simulink model "multi_model"  (R2017b)
settings: Solver=FixedStepAuto  StartTime=0.0  StopTime=10  RelTol=1e-3
undefined symbols (not defined in the file or in its folder): deg, motor_state, rad, s
libraries: simulink x7, aerolibconvert2 x4, aerolibobsolete x1, aerolibatmos2 x1, aerolibanimutils x1, aerolibnav x1
settings Model: SimulationMode=accelerator  Creator=ADAM  LastModifiedBy=moneu
settings DataIOCC: ExternalInput=initial_in  FinalStateName=final_state  InitialState=initial_state  LimitDataPoints=on  MaxDataPoints=1  LoadExternalInput=on  LoadInitialState=on  SaveFinalState=on  SaveFormat=Structure  SignalLoggingSaveFormat=ModelDataLogs  SignalLogging=off  DSMLogging=off  SaveTime=off  OutputSaveName=final_out  SignalLoggingName=model_out
settings OptimizationCC: ExpressionDepthLimit=2147483647  LifeSpan=inf
settings DebuggingCC: UnderspecifiedInitializationDetection=Classic  MergeDetectMultiDrivingBlocksExec=none  SolverPrmCheckMsg=warning  MultiTaskDSMMsg=warning  MultiTaskCondExecSysMsg=none  StateNameClashWarn=warning  StrictBusMsg=None  SFUnexpectedBacktrackingDiag=warning  SFNoUnconditionalDefaultTransitionDiag=warning  SFExecutionAtInitializationDiag=none
settings HardwareCC: ProdBitPerPointer=32  ProdBitPerSizeT=32  ProdBitPerPtrDiffT=32  ProdLargestAtomicFloat=None  ProdWordSize=32  ProdHWDeviceType=Generic->32-bit x86 compatible
settings ModelReferenceCC: UpdateModelReferenceTargets=AssumeUpToDate  CheckModelReferenceTargetMessage=none  PropagateSignalLabelsOutOfModel=off
settings RTWCC: SystemTargetFile=rtwin.tlc  TemplateMakefile=rtwin.tmf  Description=Real-Time Windows Target
settings CodeAppCC: MaxIdLength=95  StateflowObjectComments=on
settings TargetCC: TargetLibSuffix=_rtwin.lib  TargetPreCompLibLocation=C:\Program Files\MATLAB\R2013a\toolbox\rtw\targets\rtwin\lib\win64
settings ConfigComp: CovMetricSettings=dw  CovHtmlReporting=on  CovSaveCumulativeToWorkspaceVar=on  CovSaveSingleToWorkspaceVar=on  CovExternalEMLEnable=off

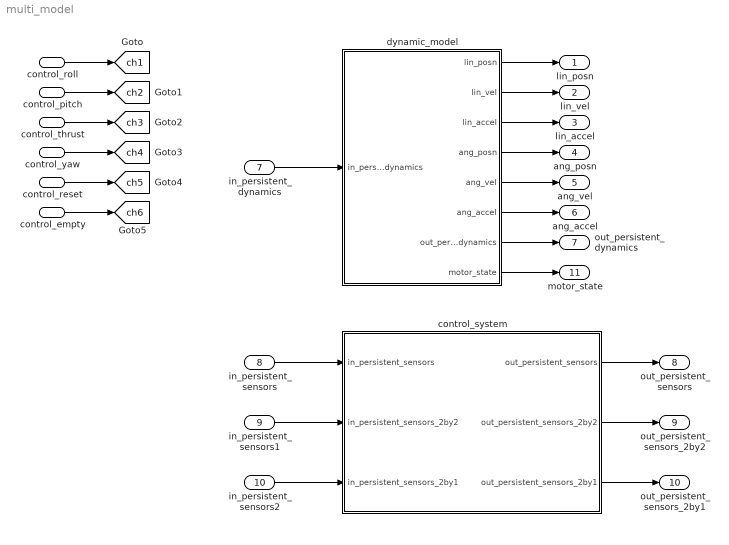
== system multi_model ==
  control_roll : Inport  PortDimensions=1
  control_pitch : Inport  Port=2  PortDimensions=1
  control_thrust : Inport  Port=3  PortDimensions=1
  control_yaw : Inport  Port=4  PortDimensions=1
  control_reset : Inport  Port=5  PortDimensions=1
  control_empty : Inport  Port=6  PortDimensions=1
  in_persistent_dynamics : Inport  Port=7  PortDimensions=1
  in_persistent_sensors : Inport  Port=8  PortDimensions=8
  in_persistent_sensors1 : Inport  Port=9  PortDimensions=[4 2]
  in_persistent_sensors2 : Inport  Port=10  PortDimensions=[2 2]
  control_system : Subsystem
  dynamic_model : Subsystem
  lin_posn : Outport
  lin_vel : Outport  Port=2
  lin_accel : Outport  Port=3
  ang_posn : Outport  Port=4
  ang_vel : Outport  Port=5
  ang_accel : Outport  Port=6
  out_persistent_dynamics : Outport  Port=7
  out_persistent_sensors : Outport  Port=8
  out_persistent_sensors_2by2 : Outport  Port=9
  out_persistent_sensors_2by1 : Outport  Port=10
  motor_state : Outport  Port=11
  tag scope: ch1=global, ch2=global, ch3=global, ch4=global, ch5=global, ch6=global
  wires:
  control_thrust/1 -> [ch3]
  control_pitch/1 -> [ch2]
  control_roll/1 -> [ch1]
  control_yaw/1 -> [ch4]
  control_reset/1 -> [ch5]
  control_empty/1 -> [ch6]
  dynamic_model/1(lin_posn) -> lin_posn/1
  dynamic_model/2(lin_vel) -> lin_vel/1
  dynamic_model/3(lin_accel) -> lin_accel/1
  dynamic_model/4(ang_posn) -> ang_posn/1
  dynamic_model/5(ang_vel) -> ang_vel/1
  dynamic_model/6(ang_accel) -> ang_accel/1
  dynamic_model/7(out_persistent_dynamics) -> out_persistent_dynamics/1
  control_system/1(out_persistent_sensors) -> out_persistent_sensors/1
  control_system/2(out_persistent_sensors_2by2) -> out_persistent_sensors_2by2/1
  control_system/3(out_persistent_sensors_2by1) -> out_persistent_sensors_2by1/1
  in_persistent_dynamics/1 -> dynamic_model/1(in_persistent_dynamics)
  in_persistent_sensors/1 -> control_system/1(in_persistent_sensors)
  in_persistent_sensors1/1 -> control_system/2(in_persistent_sensors_2by2)
  in_persistent_sensors2/1 -> control_system/3(in_persistent_sensors_2by1)
  dynamic_model/8(motor_state) -> motor_state/1

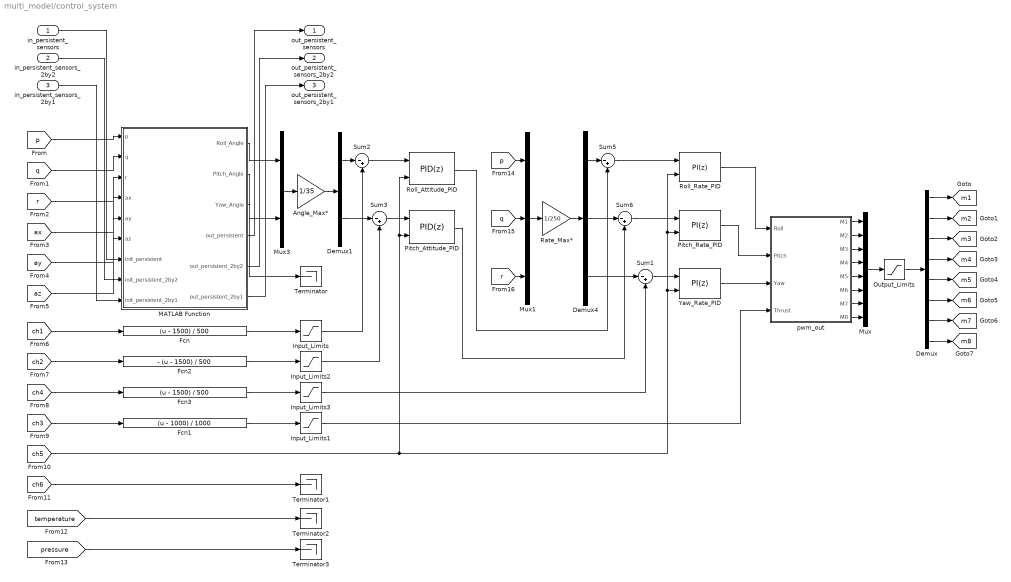
== system multi_model/control_system ==
  in_persistent_sensors : Inport
  in_persistent_sensors_2by2 : Inport  Port=2
  in_persistent_sensors_2by1 : Inport  Port=3
  Angle_Max* : Gain  Gain=1/35
  Demux : Demux  Outputs=8
  Demux1 : Demux  Outputs=2
  Demux4 : Demux  Outputs=3
  Fcn : Fcn  Expr=(u - 1500) / 500
  Fcn1 : Fcn  Expr=(u - 1000) / 1000
  Fcn2 : Fcn  Expr=- (u - 1500) / 500
  Fcn3 : Fcn  Expr=(u - 1500) / 500
  Input_Limits : Saturate  UpperLimit=1  LowerLimit=-1
  Input_Limits1 : Saturate  UpperLimit=1  LowerLimit=0
  Input_Limits2 : Saturate  UpperLimit=1  LowerLimit=-1
  Input_Limits3 : Saturate  UpperLimit=1  LowerLimit=-1
  MATLAB Function : MATLAB Function  TreatAsAtomicUnit=on
  Mux : Mux  Inputs=8
  Mux1 : Mux  Inputs=3
  Mux3 : Mux  Inputs=2
  Output_Limits : Saturate  UpperLimit=2000  LowerLimit=1000
  Pitch_Attitude_PID : simulink/Continuous/PID Controller  Controller=PID  TimeDomain=Discrete-time  SampleTime=-1  IntegratorMethod=Forward Euler  FilterMethod=Forward Euler  Form=Parallel  UseFilter=on  ControllerParametersSource=internal  P=0.8  I=0.08  D=0.08  N=100  InitialConditionSource=internal  InitialConditionForIntegrator=0  InitialConditionForFilter=0  ExternalReset=either  LimitOutput=on  UpperSaturationLimit=1  LowerSaturationLimit=-1  LinearizeAsGain=on  AntiWindupMode=none  Kb=1  TrackingMode=off  Kt=1  PParamMin=[]  PParamMax=[]  IParamMin=[]  IParamMax=[]  DParamMin=[]  DParamMax=[]  NParamMin=[]  NParamMax=[]  KbParamMin=[]  KbParamMax=[]  KtParamMin=[]  KtParamMax=[]  POutMin=[]  POutMax=[]  IOutMin=[]  IOutMax=[]  DOutMin=[]  DOutMax=[]  NOutMin=[]  NOutMax=[]  KbOutMin=[]  KbOutMax=[]  KtOutMin=[]  KtOutMax=[]  IntegratorOutMin=[]  IntegratorOutMax=[]  FilterOutMin=[]  FilterOutMax=[]  SumOutMin=[]  SumOutMax=[]  SumI1OutMin=[]  SumI1OutMax=[]  SumI2OutMin=[]  SumI2OutMax=[]  SumI3OutMin=[]  SumI3OutMax=[]  SumDOutMin=[]  SumDOutMax=[]  SaturationOutMin=[]  SaturationOutMax=[]  IntegratorContinuousStateAttributes=''  IntegratorStateMustResolveToSignalObject=off  IntegratorRTWStateStorageClass=Auto  FilterContinuousStateAttributes=''  FilterStateMustResolveToSignalObject=off  FilterRTWStateStorageClass=Auto  DifferentiatorICPrevScaledInput=0  DifferentiatorOutMin=[]  DifferentiatorOutMax=[]  InitialConditionSetting=State (most efficient)  FilterDiffOutCoefMin=[]  FilterDiffOutCoefMax=[]  SumDenOutMin=[]  SumDenOutMax=[]  SumNumOutMin=[]  SumNumOutMax=[]  ReciprocalOutMin=[]  ReciprocalOutMax=[]  DivideOutMin=[]  DivideOutMax=[]  TunerSelectOption=Transfer Function Based (PID Tuner App)
  Pitch_Rate_PID : simulink/Continuous/PID Controller  Controller=PI  TimeDomain=Discrete-time  SampleTime=-1  IntegratorMethod=Forward Euler  FilterMethod=Forward Euler  Form=Parallel  UseFilter=on  ControllerParametersSource=internal  P=1  I=0.1  D=0  N=100  InitialConditionSource=internal  InitialConditionForIntegrator=0  InitialConditionForFilter=0  ExternalReset=either  LimitOutput=on  UpperSaturationLimit=1  LowerSaturationLimit=-1  LinearizeAsGain=on  AntiWindupMode=none  Kb=1  TrackingMode=off  Kt=1  PParamMin=[]  PParamMax=[]  IParamMin=[]  IParamMax=[]  DParamMin=[]  DParamMax=[]  NParamMin=[]  NParamMax=[]  KbParamMin=[]  KbParamMax=[]  KtParamMin=[]  KtParamMax=[]  POutMin=[]  POutMax=[]  IOutMin=[]  IOutMax=[]  DOutMin=[]  DOutMax=[]  NOutMin=[]  NOutMax=[]  KbOutMin=[]  KbOutMax=[]  KtOutMin=[]  KtOutMax=[]  IntegratorOutMin=[]  IntegratorOutMax=[]  FilterOutMin=[]  FilterOutMax=[]  SumOutMin=[]  SumOutMax=[]  SumI1OutMin=[]  SumI1OutMax=[]  SumI2OutMin=[]  SumI2OutMax=[]  SumI3OutMin=[]  SumI3OutMax=[]  SumDOutMin=[]  SumDOutMax=[]  SaturationOutMin=[]  SaturationOutMax=[]  IntegratorContinuousStateAttributes=''  IntegratorStateMustResolveToSignalObject=off  IntegratorRTWStateStorageClass=Auto  FilterContinuousStateAttributes=''  FilterStateMustResolveToSignalObject=off  FilterRTWStateStorageClass=Auto  DifferentiatorICPrevScaledInput=0  DifferentiatorOutMin=[]  DifferentiatorOutMax=[]  InitialConditionSetting=State (most efficient)  FilterDiffOutCoefMin=[]  FilterDiffOutCoefMax=[]  SumDenOutMin=[]  SumDenOutMax=[]  SumNumOutMin=[]  SumNumOutMax=[]  ReciprocalOutMin=[]  ReciprocalOutMax=[]  DivideOutMin=[]  DivideOutMax=[]  TunerSelectOption=Transfer Function Based (PID Tuner App)
  Rate_Max* : Gain  Gain=1/250
  Roll_Attitude_PID : simulink/Continuous/PID Controller  Controller=PID  TimeDomain=Discrete-time  SampleTime=-1  IntegratorMethod=Forward Euler  FilterMethod=Forward Euler  Form=Parallel  UseFilter=on  ControllerParametersSource=internal  P=0.8  I=0.08  D=0.08  N=100  InitialConditionSource=internal  InitialConditionForIntegrator=0  InitialConditionForFilter=0  ExternalReset=either  LimitOutput=on  UpperSaturationLimit=1  LowerSaturationLimit=-1  LinearizeAsGain=on  AntiWindupMode=none  Kb=1  TrackingMode=off  Kt=1  PParamMin=[]  PParamMax=[]  IParamMin=[]  IParamMax=[]  DParamMin=[]  DParamMax=[]  NParamMin=[]  NParamMax=[]  KbParamMin=[]  KbParamMax=[]  KtParamMin=[]  KtParamMax=[]  POutMin=[]  POutMax=[]  IOutMin=[]  IOutMax=[]  DOutMin=[]  DOutMax=[]  NOutMin=[]  NOutMax=[]  KbOutMin=[]  KbOutMax=[]  KtOutMin=[]  KtOutMax=[]  IntegratorOutMin=[]  IntegratorOutMax=[]  FilterOutMin=[]  FilterOutMax=[]  SumOutMin=[]  SumOutMax=[]  SumI1OutMin=[]  SumI1OutMax=[]  SumI2OutMin=[]  SumI2OutMax=[]  SumI3OutMin=[]  SumI3OutMax=[]  SumDOutMin=[]  SumDOutMax=[]  SaturationOutMin=[]  SaturationOutMax=[]  IntegratorContinuousStateAttributes=''  IntegratorStateMustResolveToSignalObject=off  IntegratorRTWStateStorageClass=Auto  FilterContinuousStateAttributes=''  FilterStateMustResolveToSignalObject=off  FilterRTWStateStorageClass=Auto  DifferentiatorICPrevScaledInput=0  DifferentiatorOutMin=[]  DifferentiatorOutMax=[]  InitialConditionSetting=State (most efficient)  FilterDiffOutCoefMin=[]  FilterDiffOutCoefMax=[]  SumDenOutMin=[]  SumDenOutMax=[]  SumNumOutMin=[]  SumNumOutMax=[]  ReciprocalOutMin=[]  ReciprocalOutMax=[]  DivideOutMin=[]  DivideOutMax=[]  TunerSelectOption=Transfer Function Based (PID Tuner App)
  Roll_Rate_PID : simulink/Continuous/PID Controller  Controller=PI  TimeDomain=Discrete-time  SampleTime=-1  IntegratorMethod=Forward Euler  FilterMethod=Forward Euler  Form=Parallel  UseFilter=on  ControllerParametersSource=internal  P=1  I=0.1  D=0  N=100  InitialConditionSource=internal  InitialConditionForIntegrator=0  InitialConditionForFilter=0  ExternalReset=either  LimitOutput=on  UpperSaturationLimit=1  LowerSaturationLimit=-1  LinearizeAsGain=on  AntiWindupMode=none  Kb=1  TrackingMode=off  Kt=1  PParamMin=[]  PParamMax=[]  IParamMin=[]  IParamMax=[]  DParamMin=[]  DParamMax=[]  NParamMin=[]  NParamMax=[]  KbParamMin=[]  KbParamMax=[]  KtParamMin=[]  KtParamMax=[]  POutMin=[]  POutMax=[]  IOutMin=[]  IOutMax=[]  DOutMin=[]  DOutMax=[]  NOutMin=[]  NOutMax=[]  KbOutMin=[]  KbOutMax=[]  KtOutMin=[]  KtOutMax=[]  IntegratorOutMin=[]  IntegratorOutMax=[]  FilterOutMin=[]  FilterOutMax=[]  SumOutMin=[]  SumOutMax=[]  SumI1OutMin=[]  SumI1OutMax=[]  SumI2OutMin=[]  SumI2OutMax=[]  SumI3OutMin=[]  SumI3OutMax=[]  SumDOutMin=[]  SumDOutMax=[]  SaturationOutMin=[]  SaturationOutMax=[]  IntegratorContinuousStateAttributes=''  IntegratorStateMustResolveToSignalObject=off  IntegratorRTWStateStorageClass=Auto  FilterContinuousStateAttributes=''  FilterStateMustResolveToSignalObject=off  FilterRTWStateStorageClass=Auto  DifferentiatorICPrevScaledInput=0  DifferentiatorOutMin=[]  DifferentiatorOutMax=[]  InitialConditionSetting=State (most efficient)  FilterDiffOutCoefMin=[]  FilterDiffOutCoefMax=[]  SumDenOutMin=[]  SumDenOutMax=[]  SumNumOutMin=[]  SumNumOutMax=[]  ReciprocalOutMin=[]  ReciprocalOutMax=[]  DivideOutMin=[]  DivideOutMax=[]  TunerSelectOption=Transfer Function Based (PID Tuner App)
  Sum{1..3,5..6} (5 alike) : Sum  Inputs=|-+
  Terminator{,1..3} (4 alike) : Terminator
  Yaw_Rate_PID : simulink/Continuous/PID Controller  Controller=PI  TimeDomain=Discrete-time  SampleTime=-1  IntegratorMethod=Forward Euler  FilterMethod=Forward Euler  Form=Parallel  UseFilter=on  ControllerParametersSource=internal  P=1.5  I=0.15  D=0  N=100  InitialConditionSource=internal  InitialConditionForIntegrator=0  InitialConditionForFilter=0  ExternalReset=either  LimitOutput=on  UpperSaturationLimit=1  LowerSaturationLimit=-1  LinearizeAsGain=on  AntiWindupMode=none  Kb=1  TrackingMode=off  Kt=1  PParamMin=[]  PParamMax=[]  IParamMin=[]  IParamMax=[]  DParamMin=[]  DParamMax=[]  NParamMin=[]  NParamMax=[]  KbParamMin=[]  KbParamMax=[]  KtParamMin=[]  KtParamMax=[]  POutMin=[]  POutMax=[]  IOutMin=[]  IOutMax=[]  DOutMin=[]  DOutMax=[]  NOutMin=[]  NOutMax=[]  KbOutMin=[]  KbOutMax=[]  KtOutMin=[]  KtOutMax=[]  IntegratorOutMin=[]  IntegratorOutMax=[]  FilterOutMin=[]  FilterOutMax=[]  SumOutMin=[]  SumOutMax=[]  SumI1OutMin=[]  SumI1OutMax=[]  SumI2OutMin=[]  SumI2OutMax=[]  SumI3OutMin=[]  SumI3OutMax=[]  SumDOutMin=[]  SumDOutMax=[]  SaturationOutMin=[]  SaturationOutMax=[]  IntegratorContinuousStateAttributes=''  IntegratorStateMustResolveToSignalObject=off  IntegratorRTWStateStorageClass=Auto  FilterContinuousStateAttributes=''  FilterStateMustResolveToSignalObject=off  FilterRTWStateStorageClass=Auto  DifferentiatorICPrevScaledInput=0  DifferentiatorOutMin=[]  DifferentiatorOutMax=[]  InitialConditionSetting=State (most efficient)  FilterDiffOutCoefMin=[]  FilterDiffOutCoefMax=[]  SumDenOutMin=[]  SumDenOutMax=[]  SumNumOutMin=[]  SumNumOutMax=[]  ReciprocalOutMin=[]  ReciprocalOutMax=[]  DivideOutMin=[]  DivideOutMax=[]  TunerSelectOption=Transfer Function Based (PID Tuner App)
  pwm_out : MATLAB Function  TreatAsAtomicUnit=on
  out_persistent_sensors : Outport
  out_persistent_sensors_2by2 : Outport  Port=2
  out_persistent_sensors_2by1 : Outport  Port=3
  tag scope: m1=global, m2=global, m3=global, m4=global, m5=global, m6=global, m7=global, m8=global
  wires:
  pwm_out/8(M8) -> Mux/8
  pwm_out/7(M7) -> Mux/7
  pwm_out/6(M6) -> Mux/6
  pwm_out/5(M5) -> Mux/5
  pwm_out/4(M4) -> Mux/4
  pwm_out/3(M3) -> Mux/3
  pwm_out/2(M2) -> Mux/2
  pwm_out/1(M1) -> Mux/1
  Sum5/1 -> Roll_Rate_PID/1
  Rate_Max*/1 -> Demux4/1
  Demux4/2 -> Sum6/1
  Demux4/1 -> Sum5/1
  Sum1/1 -> Yaw_Rate_PID/1
  Sum6/1 -> Pitch_Rate_PID/1
  Demux4/3 -> Sum1/1
  Mux1/1 -> Rate_Max*/1
  Roll_Rate_PID/1 -> pwm_out/1(Roll)
  Pitch_Rate_PID/1 -> pwm_out/2(Pitch)
  Yaw_Rate_PID/1 -> pwm_out/3(Yaw)
  Mux3/1 -> Angle_Max*/1
  Sum2/1 -> Roll_Attitude_PID/1
  Sum3/1 -> Pitch_Attitude_PID/1
  Angle_Max*/1 -> Demux1/1
  Demux1/2 -> Sum3/1
  Demux1/1 -> Sum2/1
  Pitch_Attitude_PID/1 -> Sum6/2
  Roll_Attitude_PID/1 -> Sum5/2
  Input_Limits2/1 -> Sum3/2
  Input_Limits3/1 -> Sum1/2
  Input_Limits/1 -> Sum2/2
  Demux/1 -> [m1]
  Demux/2 -> [m2]
  Demux/3 -> [m3]
  Demux/4 -> [m4]
  Demux/5 -> [m5]
  Demux/6 -> [m6]
  Demux/7 -> [m7]
  Demux/8 -> [m8]
  Mux/1 -> Output_Limits/1
  Output_Limits/1 -> Demux/1
  Fcn1/1 -> Input_Limits1/1
  Input_Limits1/1 -> pwm_out/4(Thrust)
  Fcn2/1 -> Input_Limits2/1
  Fcn3/1 -> Input_Limits3/1
  [ch3] -> Fcn1/1
  [ch4] -> Fcn3/1
  [ch2] -> Fcn2/1
  [ch1] -> Fcn/1
  [ch5] -> Roll_Rate_PID/2, Pitch_Rate_PID/2, Yaw_Rate_PID/2, Roll_Attitude_PID/2, Pitch_Attitude_PID/2
  Fcn/1 -> Input_Limits/1
  [ch6] -> Terminator1/1
  MATLAB Function/3(Yaw_Angle) -> Terminator/1
  MATLAB Function/2(Pitch_Angle) -> Mux3/2
  MATLAB Function/1(Roll_Angle) -> Mux3/1
  [ax] -> MATLAB Function/4(ax)
  [ay] -> MATLAB Function/5(ay)
  [az] -> MATLAB Function/6(az)
  [r] -> MATLAB Function/3(r)
  [q] -> MATLAB Function/2(q)
  [p] -> MATLAB Function/1(p)
  [pressure] -> Terminator3/1
  [temperature] -> Terminator2/1
  [p] -> Mux1/1
  [q] -> Mux1/2
  [r] -> Mux1/3
  in_persistent_sensors/1 -> MATLAB Function/7(init_persistent)
  MATLAB Function/4(out_persistent) -> out_persistent_sensors/1
  in_persistent_sensors_2by2/1 -> MATLAB Function/8(init_persistent_2by2)
  in_persistent_sensors_2by1/1 -> MATLAB Function/9(init_persistent_2by1)
  MATLAB Function/5(out_persistent_2by2) -> out_persistent_sensors_2by2/1
  MATLAB Function/6(out_persistent_2by1) -> out_persistent_sensors_2by1/1

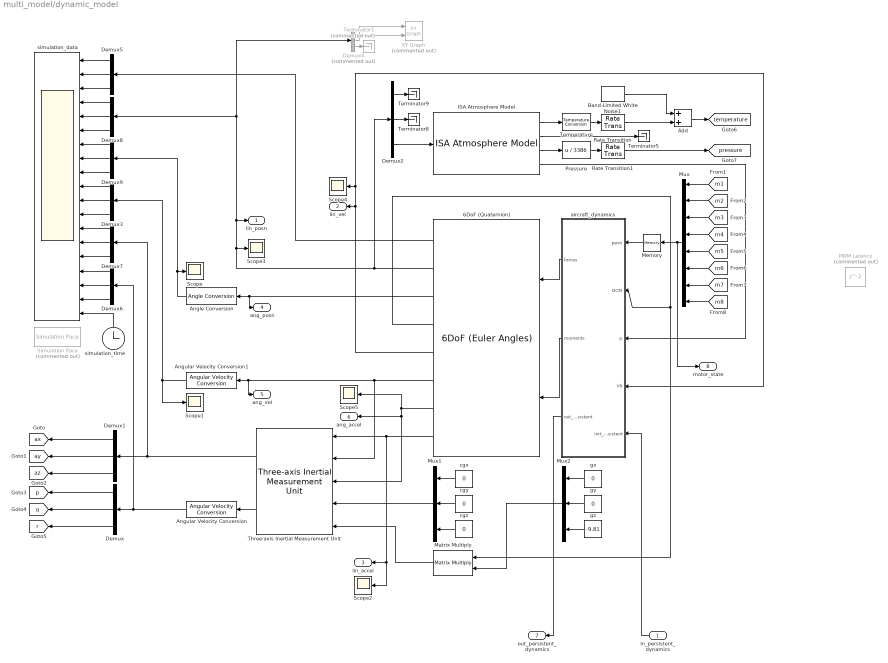
== system multi_model/dynamic_model ==
  in_persistent_dynamics : Inport
  6DoF (Quaternion) : aerolibobsolete/6DoF (Euler Angles)  units=Metric (MKS)  mtype=Fixed  rep=Quaternion  xme_0=[0 0 0]  Vm_0=[0 0 0]  eul_0=[0 0 0]  pm_0=[0 0 0]  mass_0=1  mass_e=0  mass_f=0  inertia=[0.016, 0, 0; 0, 0.016, 0; 0, 0, 0.031]  inertia_e=eye(3)  inertia_f=eye(3)  k_quat=1.0
      settings: SourceProductName=Aerospace Blockset  SourceProductBaseCode=AE
  Add : Sum
  Angle Conversion : aerolibconvert2/Angle Conversion  IU=rad  OU=deg
  Angular Velocity Conversion : aerolibconvert2/Angular Velocity Conversion  IU=rad/s  OU=deg/s
      settings: SourceProductName=Aerospace Blockset
  Angular Velocity Conversion1 : aerolibconvert2/Angular Velocity Conversion  IU=rad/s  OU=deg/s
      settings: SourceProductName=Aerospace Blockset
  Band-Limited White Noise1 : simulink/Sources/Band-Limited White Noise  Cov=[0.0001]  Ts=0.5  seed=[23341]
  Demux{,1..3,5..9} (9 alike) : Demux  Outputs=3
  Demux4 : Demux  Commented=on  Outputs=3
  ISA Atmosphere Model : aerolibatmos2/ISA Atmosphere Model  custom=on  g=9.80665  gamma=1.4  R=287.0531  L=0.0065  h_trop=11000  h_strat=20000  rho0=1.225  P0=101325  T0=288.15  h0=0
      settings: SourceProductName=Aerospace Blockset
  Matrix Multiply : Product  Multiplication=Matrix(*)
  Memory : Memory  InitialCondition=motor_state
  Mux : Mux  Inputs=8
  Mux1 : Mux  Inputs=3
  Mux2 : Mux  Inputs=3
  PWM Latency : Delay  Commented=on
  Pressure : Fcn  Expr=u / 3386
  Rate Transition : RateTransition  OutPortSampleTime=0.01
  Rate Transition1 : RateTransition  OutPortSampleTime=0.05
  Scope{,1..5} (6 alike) : Scope
  Simulation Pace : aerolibanimutils/Simulation Pace  Commented=on  SimulationPace=1  SleepMode=MATLAB Thread  OutputPaceError=off  SampleTime=-1
      settings: AttributesFormatString=%<SimulationPace> sec/sec
  Temperature : aerolibconvert2/Temperature Conversion  IU=K  OU=C
      settings: SourceProductName=Aerospace Blockset  SourceProductBaseCode=AE
  Terminator1 : Terminator  Commented=on
  Terminator5 : Terminator
  Terminator8 : Terminator
  Terminator9 : Terminator
  Three-axis Inertial Measurement Unit : aerolibnav/Three-axis Inertial Measurement Unit  units=Metric (MKS)  imu=[0 0 0]  i_Ts=0.01  dtype_a=off  w_a=190  z_a=0.707  a_sf_cc=[0.98 0 0; 0 0.98 0; 0 0 -0.98]  a_bias=[0 0 0]  a_sat="[-19.62  -19.62  -19.62 19.62 19.62 19.62]"  dtype_g=off  w_g=190  z_g=0.707  g_sf_cc=[.98 0 0; 0 .98 0; 0 0 .98]  g_bias=[0 0 0]  g_sens=[0 0 0]  g_sat="[-4.36  -4.36  -4.36 4.36 4.36 4.36]"  i_rand=on  i_seeds=[348631 366719 978432 189621 128794 214632]  i_pow=[0.000039 0.000039 0.000039 0.000000087 0.000000087 0.000000087]
  XY Graph : simulink/Sinks/XY Graph  Commented=on  xmin=-10  xmax=10  ymin=-10  ymax=10  st=-1
  aircraft_dynamics : MATLAB Function  TreatAsAtomicUnit=on
  cgx : Constant  Value=0
  cgy : Constant  Value=0
  cgz : Constant  Value=0
  gx : Constant  Value=0
  gy : Constant  Value=0
  gz : Constant  Value=-9.81
  simulation_data : Scope  NumInputPorts=19
  simulation_time : Clock
  lin_posn : Outport
  lin_vel : Outport  Port=2
  lin_accel : Outport  Port=3
  ang_posn : Outport  Port=4
  ang_vel : Outport  Port=5
  ang_accel : Outport  Port=6
  out_persistent_dynamics : Outport  Port=7
  motor_state : Outport  Port=8
  tag scope: ax=global, ay=global, az=global, p=global, pressure=global, q=global, r=global, temperature=global
  wires:
  Three-axis Inertial Measurement Unit/2 -> Angular Velocity Conversion/1
  cgy/1 -> Mux1/2
  cgx/1 -> Mux1/1
  cgz/1 -> Mux1/3
  Mux1/1 -> Three-axis Inertial Measurement Unit/4
  6DoF (Quaternion)/7 -> ang_accel/1, Three-axis Inertial Measurement Unit/3, Scope5/1
  [m1] -> Mux/1
  [m3] -> Mux/3
  Demux1/1 -> [ax]
  [m2] -> Mux/2
  [m6] -> Mux/6
  [m5] -> Mux/5
  [m8] -> Mux/8
  [m4] -> Mux/4
  [m7] -> Mux/7
  6DoF (Quaternion)/8 -> lin_accel/1, Scope2/1, Three-axis Inertial Measurement Unit/1
  6DoF (Quaternion)/4 -> Matrix Multiply/1, aircraft_dynamics/2(DCM)
  gy/1 -> Mux2/2
  gx/1 -> Mux2/1
  gz/1 -> Mux2/3
  Demux2/2 -> Terminator8/1
  Demux2/1 -> Terminator9/1
  Demux2/3 -> ISA Atmosphere Model/1
  6DoF (Quaternion)/2 -> Demux2/1, Demux4/1, Demux8/1, lin_posn/1, Scope3/1
  ISA Atmosphere Model/3 -> Pressure/1
  ISA Atmosphere Model/2 -> Terminator5/1
  ISA Atmosphere Model/4 -> aircraft_dynamics/3(p)
  6DoF (Quaternion)/5 -> lin_vel/1, Scope4/1, aircraft_dynamics/4(Vb)
  Demux1/3 -> [az]
  ISA Atmosphere Model/1 -> Temperature/1
  Temperature/1 -> Rate Transition/1
  aircraft_dynamics/2(moments) -> 6DoF (Quaternion)/2
  Mux2/1 -> Matrix Multiply/2
  Matrix Multiply/1 -> Three-axis Inertial Measurement Unit/5
  aircraft_dynamics/1(forces) -> 6DoF (Quaternion)/1
  Demux9/1 -> simulation_data/7
  Demux9/2 -> simulation_data/8
  Demux3/1 -> simulation_data/10
  Demux3/2 -> simulation_data/11
  Demux3/3 -> simulation_data/12
  Demux7/1 -> simulation_data/13
  Demux7/2 -> simulation_data/14
  Demux7/3 -> simulation_data/15
  Angle Conversion/1 -> Demux9/1, Scope/1
  Demux/1 -> [p]
  Demux/2 -> [q]
  Demux/3 -> [r]
  Demux1/2 -> [ay]
  Demux5/1 -> simulation_data/1
  Demux5/2 -> simulation_data/2
  Demux5/3 -> simulation_data/3
  Demux8/1 -> simulation_data/4
  Demux8/2 -> simulation_data/5
  Demux8/3 -> simulation_data/6
  6DoF (Quaternion)/6 -> Three-axis Inertial Measurement Unit/2, ang_vel/1, Angular Velocity Conversion1/1
  Demux9/3 -> simulation_data/9
  Demux6/1 -> simulation_data/16
  Demux6/2 -> simulation_data/17
  Demux6/3 -> simulation_data/18
  simulation_time/1 -> simulation_data/19
  Pressure/1 -> Rate Transition1/1
  Rate Transition/1 -> Add/2
  Add/1 -> [temperature]
  Rate Transition1/1 -> [pressure]
  Band-Limited White Noise1/1 -> Add/1
  6DoF (Quaternion)/1 -> Demux5/1
  Three-axis Inertial Measurement Unit/1 -> Demux7/1, Demux1/1
  Angular Velocity Conversion/1 -> Demux/1, Demux6/1
  6DoF (Quaternion)/3 -> ang_posn/1, Angle Conversion/1
  Angular Velocity Conversion1/1 -> Scope1/1, Demux3/1
  Mux/1 -> motor_state/1, Memory/1
  Memory/1 -> aircraft_dynamics/1(pwm)
  Demux4/1 -> XY Graph/2
  Demux4/2 -> XY Graph/1
  Demux4/3 -> Terminator1/1
  aircraft_dynamics/3(out_persistent) -> out_persistent_dynamics/1
  in_persistent_dynamics/1 -> aircraft_dynamics/5(init_persistent)

== matlab function multi_model/control_system/MATLAB Function ==
  data: p input; Roll_Angle output; q input; r input; ax input; ay input; az input; Pitch_Angle output; Yaw_Angle output; init_persistent input; out_persistent output; init_persistent_2by2 input; init_persistent_2by1 input; out_persistent_2by2 output; out_persistent_2by1 output
function [Roll_Angle, Pitch_Angle, Yaw_Angle, out_persistent, out_persistent_2by2, out_persistent_2by1] = sensor_fusion(p, q, r, ax, ay, az, init_persistent, init_persistent_2by2, init_persistent_2by1)

%================================Constants=================================

delta_t = 0.01;
degrees = 180 / pi;
radians = pi / 180;

%Attitude Estimator
Q_gyroBias = 0.000000087;           % Q_gyroBias: gyroscope noise
Q_angle = 0.000039;                 % Q_angle: accelerometer noise
R_angle = 20;                       % R_angle: high ==> gyroscope, low ==> accelerometer

%=============================Intitialization==============================

persistent initialize angle_roll bias1 P1 K1 phi angle_pitch bias2 P2 K2 theta angle_yaw;
    
if isempty(initialize)
    if ~init_persistent(1)
        if isempty(angle_roll)
            angle_roll = 0;
            bias1 = 0;
            P1 = zeros(2);
            K1 = zeros([2,1]);
            phi = 0;
        end
        if isempty(angle_pitch)
            angle_pitch = 0;
            bias2 = 0;
            P2 = zeros(2);
            K2 = zeros([2,1]);
            theta = 0;
        end
        if isempty(angle_yaw)
            angle_yaw = 0;
        end
        initialize = 1;
    else
        initialize = init_persistent(1);
        angle_roll = init_persistent(2);
        bias1 = init_persistent(3);
        phi = init_persistent(4);
        angle_pitch = init_persistent(5);
        bias2 = init_persistent(6);
        theta = init_persistent(7);
        angle_yaw = init_persistent(8);
        P1 = init_persistent_2by2(1:2,:);
        P2 = init_persistent_2by2(3:4,:);
        K1 = init_persistent_2by1(:,1);
        K2 = init_persistent_2by1(:,2);
    end
else
    
%==============================Kalman Filter===============================

%--------------------------------Roll Angle--------------------------------

    Rate_Roll = p + (q * sin(phi) + r * cos(phi)) * tan(theta) - bias1;                     
    angle_roll = angle_roll + Rate_Roll * delta_t;                                          %Projected State (integrated gyro data)
    earth_roll = -atan(ay / az) * degrees;                                                  %Measurement Update (gravity vector)
    P1(1,1) = P1(1,1) + delta_t * (P1(2,2) * delta_t - P1(1,2) - P1(2,1) + Q_angle);        %Projected error covariance
    P1(1,2) = P1(1,2) - P1(2,2) * delta_t;
    P1(2,1) = P1(2,1) - P1(2,2) * delta_t;
    P1(2,2) = P1(2,2) + Q_gyroBias * delta_t;
    S1 = P1(1,1) + R_angle;                                                                 %Kalman Gain
    K1(1) = P1(1,1) / S1;
    K1(2) = P1(2,1) / S1;
    Y1 = earth_roll - angle_roll;                                                           %Estimate Update
    angle_roll = angle_roll + K1(1) * Y1;
    bias1 = bias1 + K1(2) * Y1;
    P1(1,1) = P1(1,1) - K1(1) * P1(1,1);                                                    %Update Error Covariance
    P1(1,2) = P1(1,2) - K1(1) * P1(1,2);
    P1(2,1) = P1(2,1) - K1(2) * P1(1,1);
    P1(2,2) = P1(2,2) - K1(2) * P1(1,2);
    phi = angle_roll * radians;
 
%--------------------------------Pitch Angle-------------------------------

    Rate_Pitch = q * cos(phi) + r * sin(phi) - bias2;                           
    angle_pitch = angle_pitch + Rate_Pitch * delta_t;                                       %Projected State (integrated gyro data)
    earth_pitch = atan(ax / az) * degrees;                                                  %Measurement Update (gravity vector)
    P2(1,1) = P2(1,1) + delta_t * (P2(2,2) * delta_t - P2(1,2) - P2(2,1) + Q_angle);        %Projected error covariance
    P2(1,2) = P2(1,2) - P2(2,2) * delta_t;
    P2(2,1) = P2(2,1) - P2(2,2) * delta_t;
    P2(2,2) = P2(2,2) + Q_gyroBias * delta_t;
    S2 = P2(1,1) + R_angle;                                                                 %Kalman Gain
    K2(1) = P2(1,1) / S2;
    K2(2) = P2(2,1) / S2;
    Y2 = earth_pitch - angle_pitch;                                                         %Estimate Update
    angle_pitch = angle_pitch + K2(1) * Y2;
    bias2 = bias2 + K2(2) * Y2;
    P2(1,1) = P2(1,1) - K2(1) * P2(1,1);                                                    %Update Error Covariance
    P2(1,2) = P2(1,2) - K2(1) * P2(1,2);
    P2(2,1) = P2(2,1) - K2(2) * P2(1,1);
    P2(2,2) = P2(2,2) - K2(2) * P2(1,2);
    theta = angle_pitch * radians;
    
%--------------------------------Yaw Angle---------------------------------

    angle_yaw = angle_yaw + (q * sin(phi) + r * cos(phi)) * sec(theta) * delta_t;           %Integrated gyro data

end

Roll_Angle = angle_roll;
Pitch_Angle = angle_pitch;
Yaw_Angle = angle_yaw;
    
%==========================================================================
out_persistent = [initialize angle_roll bias1 phi angle_pitch bias2 theta angle_yaw];
out_persistent_2by2 = zeros(4,2);
out_persistent_2by2(1:2,:) = P1;
out_persistent_2by2(3:4,:) = P2;
out_persistent_2by1 = zeros(2,2);
out_persistent_2by1(:,1) = K1;
out_persistent_2by1(:,2) = K2;

== matlab function multi_model/dynamic_model/aircraft_dynamics ==
  settings: updateMethod=DISCRETE
  data: pwm input; forces output; moments output; DCM input; p input; Vb input; init_persistent input; out_persistent output
function [forces, moments, out_persistent] = dynamics(pwm, DCM, p, Vb, init_persistent)

%================================Constants=================================

radsec = 0.104719755;
gravity = 9.81;
radians = pi / 180;

% Aircraft Parameters
motor_thrust = 0.5;                 % Maximum thrust of a single motor      (kg)
motor_constant = 880;               % Motor revolutions per volt            (KV)
motor_voltage = 11.1;               % Nominal motor voltage                 (V)
motor_efficiency = 0.8;             % Effective velocity
rotor_diameter = 0.25;              % Diameter of the rotor                 (meters)                                 
aircraft_mass = 1.0;                % Aircraft mass                         (kg)                                        
aircraft_diameter = 0.50;           % Motor to motor distance               (meters)                                      
aircraft_dihedral = 0.01;              % Angle from base to arm                (degrees)
aircraft_mixer = 0;                 % Rotor position and rotation      
                                        % Quad [X] = 0
                                        % Quad [+] = 1
                                        % Hex  [X] = 2
                                        
%==============================Inertia Tensor==============================
                                    
% 3DR Quad - 1.0kg, Standard Motor  [0.016, 0, 0; 0, 0.016, 0; 0, 0, 0.031]
% MiniQuad - 0.7kg, Mini Motor    [0.0047, 0, 0; 0.0000043, 0.0044, 0; 0.0000074, 0.0000012, 0.0086]

%==============================Initialization==============================

persistent initialize;

g = [0; 0; gravity];
t = zeros(1, 8);

if isempty(initialize)
    if ~init_persistent
        DCM = zeros(3);
        initialize = 1;
    else
        
        initialize = init_persistent;
    end
end

for n = 1:8
    t(n) = (pwm(n) - 1000) / 1000;
end
       
%=================================Actuators================================

% [enabled, x(roll), y(pitch), z(yaw)]

M = zeros(8, 4);

if aircraft_mixer == 0
    M(1, :) = [1;  1;  1; -1];
    M(2, :) = [1, -1,  1,  1];
    M(3, :) = [1, -1, -1, -1];
    M(4, :) = [1,  1, -1,  1];
    M(5, :) = [0,  0,  0,  0];
    M(6, :) = [0,  0,  0,  0];
    M(7, :) = [0,  0,  0,  0];
    M(8, :) = [0,  0,  0,  0];
elseif aircraft_mixer == 1
    M(1, :) = [1;  0;  1; -1];
    M(2, :) = [1, -1,  0,  1];
    M(3, :) = [1,  0, -1, -1];
    M(4, :) = [1,  1,  0,  1];
    M(5, :) = [0,  0,  0,  0];
    M(6, :) = [0,  0,  0,  0];
    M(7, :) = [0,  0,  0,  0];
    M(8, :) = [0,  0,  0,  0];
elseif aircraft_mixer == 2
    M(1, :) = [1;  1;  1; -1];
    M(2, :) = [1, -1,  1,  1];
    M(3, :) = [1, -1,  0, -1];
    M(4, :) = [1, -1, -1,  1];
    M(5, :) = [1,  1, -1, -1];
    M(6, :) = [1,  1,  0,  1];
    M(7, :) = [0,  0,  0,  0];
    M(8, :) = [0,  0,  0,  0];
else
    M(1, :) = [0;  0;  0;  0];
    M(2, :) = [0,  0,  0,  0];
    M(3, :) = [0,  0,  0,  0];
    M(4, :) = [0,  0,  0,  0];
    M(5, :) = [0,  0,  0,  0];
    M(6, :) = [0,  0,  0,  0];
    M(7, :) = [0,  0,  0,  0];
    M(8, :) = [0,  0,  0,  0];
end

%==================================Forces==================================

F_z = zeros(1, 8);

for n = 1:8
    F_z(n) = t(n) * motor_thrust * gravity * M(n, 1)...                     % rotor forces
    * sin((90 - aircraft_dihedral) * radians);                         
end

A = [rotor_diameter * 0.01,...                                              % rotor cross sectional area
    aircraft_diameter ^ 2 / 10,...                                          % body cross sectional area (X)
    aircraft_diameter ^ 2 / 10,...                                          % body cross sectional area (Y)
    pi * ((aircraft_diameter - rotor_diameter) / 2) ^ 2];                   % body cross sectional area (Z)

F_d = zeros(1, 3);

for n = 1:3
    F_d(n) = p / 2 * A(n + 1) * (Vb(n)) ^ 2;
    if Vb(n) > 0
        F_d(n) = F_d(n) * -1;
    end
end

forces = zeros(3, 1);

F_g = aircraft_mass .* (DCM * g);                                           % gravitational force
forces(1) = F_g(1) + F_d(1);
forces(2) = F_g(2) + F_d(2);
forces(3) = F_g(3) - sum(F_z) + 2 * F_d(3);

%==================================Moments=================================

m = zeros(8, 4);

for n = 1:8
    m(n, :) = F_z(n) .* M(n, :);
end

m = (aircraft_diameter / 2) .* m;                                           % x & y moments

K = motor_constant * motor_voltage * motor_efficiency * radsec;
Vr = zeros(1, 8);

for n = 1:8    
    Vr(n) = t(n) * K;                                                       % rotor angular velocity
end

d = zeros(1, 8);

for n = 1:8
    d(n) =  M(n, 4) * p / 2 * A(1) * (Vr(n) * rotor_diameter / 10) ^ 2;     % aerodynamic drag force of the rotor
end

T = zeros(1, 8);

for n = 1:8
    T(n) = d(n);                                                            % total rotor torque
end

moments = zeros(3, 1);

moments(1) = sum(m(:, 2));
moments(2) = sum(m(:, 3));
moments(3) = sum(T); 

%==========================================================================

out_persistent = initialize;

== matlab function multi_model/control_system/pwm_out ==
  data: Roll input; M1 output; Pitch input; Yaw input; Thrust input; M2 output; M3 output; M4 output; M5 output; M6 output; M7 output; M8 output
function [M1, M2, M3, M4, M5, M6, M7, M8] = motor_mixer(Roll, Pitch, Yaw, Thrust)

%===========================Settings & Constants===========================

idle_PWM = 1000;
aircraft_mixer = 0;  
                    % Quad [X] = 0
                    % Quad [+] = 1
                    % Hex  [X] = 2

%===============================Quad X Mixer===============================
  
if aircraft_mixer == 0        % Quad X
    M1 = ((Roll + Pitch - Yaw) * Thrust / 2 + Thrust) * 1000 + idle_PWM;
    M2 = ((-Roll + Pitch + Yaw) * Thrust / 2 + Thrust) * 1000 + idle_PWM;
    M3 = ((-Roll - Pitch - Yaw) * Thrust / 2 + Thrust) * 1000 + idle_PWM;
    M4 = ((Roll - Pitch + Yaw) * Thrust / 2 + Thrust) * 1000 + idle_PWM;
    M5 = 1000;
    M6 = 1000;
    M7 = 1000;
    M8 = 1000;
elseif aircraft_mixer == 1    % Quad +
    M1 = ((Pitch - Yaw) * Thrust / 2 + Thrust) * 1000 + idle_PWM;
    M2 = ((-Roll + Yaw) * Thrust / 2 + Thrust) * 1000 + idle_PWM;
    M3 = ((-Pitch - Yaw) * Thrust / 2 + Thrust) * 1000 + idle_PWM;
    M4 = ((Roll + Yaw) * Thrust / 2 + Thrust) * 1000 + idle_PWM;
    M5 = 1000;
    M6 = 1000;
    M7 = 1000;
    M8 = 1000;
elseif aircraft_mixer == 2    % Hex X
    M1 = ((Pitch + Roll / 2 - Yaw) * Thrust / 2 + Thrust) * 1000 + idle_PWM;
    M2 = ((Pitch - Roll / 2 + Yaw) * Thrust / 2 + Thrust) * 1000 + idle_PWM;
    M3 = ((-Roll - Yaw) * Thrust / 2 + Thrust) * 1000 + idle_PWM;
    M4 = ((-Pitch - Roll / 2 + Yaw) * Thrust / 2 + Thrust) * 1000 + idle_PWM;
    M5 = ((-Pitch + Roll / 2 - Yaw) * Thrust / 2 + Thrust) * 1000 + idle_PWM;
    M6 = ((Roll + Yaw) * Thrust / 2 + Thrust) * 1000 + idle_PWM;
    M7 = 1000;
    M8 = 1000;
else
    M1 = 1000;
    M2 = 1000;
    M3 = 1000;
    M4 = 1000;
    M5 = 1000;
    M6 = 1000;
    M7 = 1000;
    M8 = 1000;
end
%==========================================================================
